simulink model "modelh"  (R2019b)
settings: Solver=VariableStepAuto  StartTime=0.0  StopTime=10.0  RelTol=1e-3
values from neighbouring files (symbols this model uses):
  alphaH = 1-exp(-1/d_Hj)    [parameters.m]
  alphaI = 1-exp(-d_Is)    [parameters.m]
  alphaJ = 1-exp(-1/d_J)    [parameters.m]
  beta_h = 0.66    [parameters.m]
  beta_l = 0.01    [parameters.m]
  c = 2    [parameters.m]
  gammaA = 1-exp(-1/d_Ia)    [parameters.m]
  gammaH = 1-exp(-1/d_Hr)    [parameters.m]
  gammaZ = 1-exp(-1/d_Iz)    [parameters.m]
  p_d_mu = 0.49    [parameters.m]
  p_d_sd = 0.1    [parameters.m]
  p_h = 0.055    [parameters.m]
  p_j_mu = 0.23    [parameters.m]
  p_j_sd = 0.1    [parameters.m]
  p_s_h = 0.99    [parameters.m]
  p_s_l = 0.5    [parameters.m]
  psi = 1-exp(-1/d_Ip)    [parameters.m]
  r_beta_h = 0.99    [parameters.m]
  r_beta_l = 0.4    [parameters.m]
  r_c_h = 0.5    [parameters.m]
  r_c_l = 0.01    [parameters.m]
  sigma = 1 - exp(-1/d_E)    [parameters.m]
settings Model: Creator=Viktor  LastModifiedBy=Viktor

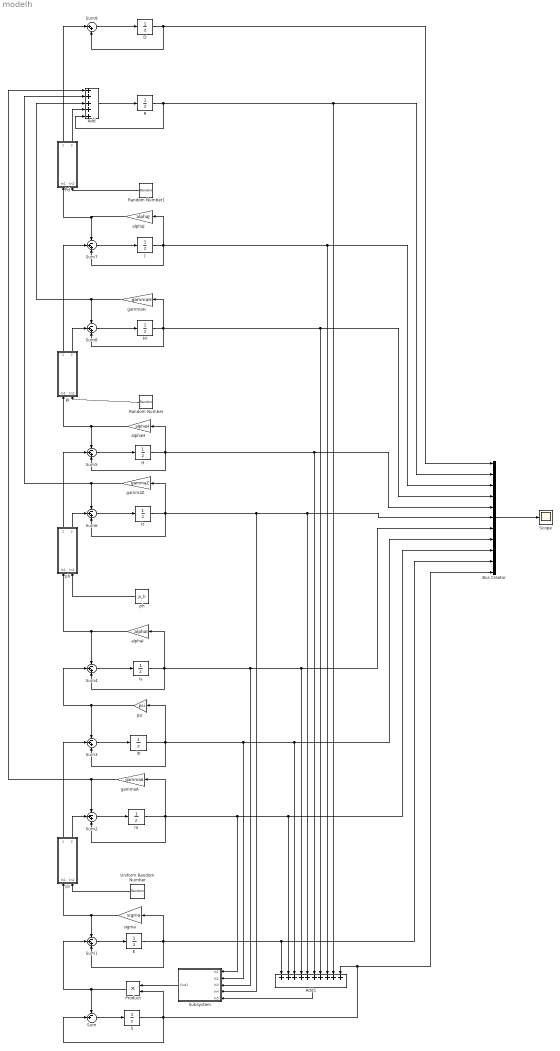
== system modelh ==
  Add : Sum  Inputs=+++++
  Add1 : Sum  Inputs=++++++++++
  Bus Creator : BusCreator  Inputs=11
  D : UnitDelay  SampleTime=-1  HasFrameUpgradeWarning=on
  E : UnitDelay  InitialCondition=10000  SampleTime=-1  HasFrameUpgradeWarning=on
  H : UnitDelay  InitialCondition=5000  SampleTime=-1  HasFrameUpgradeWarning=on
  Hr : UnitDelay  InitialCondition=5000  SampleTime=-1  HasFrameUpgradeWarning=on
  Ia : UnitDelay  InitialCondition=5000  SampleTime=-1  HasFrameUpgradeWarning=on
  Ip : UnitDelay  InitialCondition=5000  SampleTime=-1  HasFrameUpgradeWarning=on
  Is : UnitDelay  InitialCondition=5000  SampleTime=-1  HasFrameUpgradeWarning=on
  Iz : UnitDelay  InitialCondition=5000  SampleTime=-1  HasFrameUpgradeWarning=on
  J : UnitDelay  InitialCondition=5000  SampleTime=-1  HasFrameUpgradeWarning=on
  Pd : Subsystem
  Product : Product
  R : UnitDelay  InitialCondition=5000  SampleTime=-1  HasFrameUpgradeWarning=on
  Random Number : RandomNumber  Mean=p_j_mu  Variance=p_j_sd  SampleTime=0.1
  Random Number1 : RandomNumber  Mean=p_d_mu  Variance=p_d_sd  SampleTime=0.1
  S : UnitDelay  InitialCondition=5000000  SampleTime=-1  HasFrameUpgradeWarning=on
  Scope : Scope
  Subsystem : Subsystem
  Sum : Sum  Inputs=-+|
  Sum{1..8} (8 alike) : Sum  Inputs=-++
  Sum9 : Sum  Inputs=|++
  Uniform Random Number : UniformRandomNumber  Minimum=p_s_l  Maximum=p_s_h  SampleTime=0.1
  alphaH : Gain  Gain=alphaH
  alphaI : Gain  Gain=alphaI
  alphaJ : Gain  Gain=alphaJ
  gammaA : Gain  Gain=gammaA
  gammaH : Gain  Gain=gammaH
  gammaZ : Gain  Gain=gammaZ
  ph : Subsystem
  "ph " : Constant  Value=p_h
  pj : Subsystem
  "ps " : Subsystem
  psi : Gain  Gain=psi
  sigma : Gain  Gain=sigma
  wires:
  S/1 -> Product/2, Bus Creator/11, Add1/10, Sum/2
  Sum/1 -> S/1
  Product/1 -> Sum1/2, Sum/1
  Sum1/1 -> E/1
  sigma/1 -> Sum1/1, "ps "/1(In1)
  Uniform Random Number/1 -> "ps "/2(In2)
  "ps "/2(Out2) -> Sum2/2
  Sum2/1 -> Ia/1
  Ia/1 -> Subsystem/1(In1), Bus Creator/9, Add1/2, gammaA/1, Sum2/3
  Sum3/1 -> Ip/1
  Ip/1 -> Subsystem/2(In2), Bus Creator/8, Add1/3, psi/1, Sum3/3
  "ps "/1(Out1) -> Sum3/2
  psi/1 -> Sum4/2, Sum3/1
  Sum4/1 -> Is/1
  Is/1 -> Subsystem/3(In3), Bus Creator/7, Add1/4, alphaI/1, Sum4/3
  alphaI/1 -> ph/1(In1), Sum4/1
  "ph "/1 -> ph/2(In2)
  Sum5/1 -> H/1
  alphaH/1 -> pj/1(In1), Sum5/1
  Sum6/1 -> Iz/1
  Iz/1 -> Add1/5, Bus Creator/6, Subsystem/4(In4), gammaZ/1, Sum6/3
  ph/2(Out2) -> Sum6/2
  gammaZ/1 -> Add/2, Sum6/1
  Sum7/1 -> J/1
  Random Number/1 -> pj/2(In2)
  pj/1(Out1) -> Sum7/2
  Sum8/1 -> Hr/1
  pj/2(Out2) -> Sum8/2
  gammaH/1 -> Sum8/1, Add/3
  alphaJ/1 -> Pd/1(In1), Sum7/1
  Random Number1/1 -> Pd/2(In2)
  Pd/1(Out1) -> Sum9/1
  Sum9/1 -> D/1
  D/1 -> Sum9/2, Bus Creator/1
  Add/1 -> R/1
  Pd/2(Out2) -> Add/4
  ph/1(Out1) -> Sum5/2
  gammaA/1 -> Sum2/1, Add/1
  Add1/1 -> Subsystem/5(In5)
  Subsystem/1(Out1) -> Product/1
  R/1 -> Bus Creator/2, Add1/9, Add/5
  J/1 -> Add1/8, Bus Creator/3, alphaJ/1, Sum7/3
  Hr/1 -> Add1/7, Bus Creator/4, gammaH/1, Sum8/3
  H/1 -> Add1/6, Bus Creator/5, alphaH/1, Sum5/3
  E/1 -> Bus Creator/10, Add1/1, sigma/1, Sum1/3
  Bus Creator/1 -> Scope/1

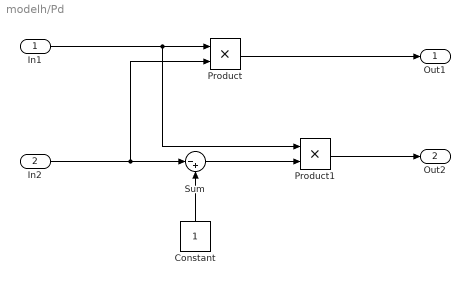
== system modelh/Pd ==
  In1 : Inport
  In2 : Inport  Port=2
  Constant : Constant
  Product : Product
  Product1 : Product
  Sum : Sum  Inputs=|-+
  Out1 : Outport
  Out2 : Outport  Port=2
  wires:
  In1/1 -> Product1/1, Product/1
  Product/1 -> Out1/1
  In2/1 -> Sum/1, Product/2
  Constant/1 -> Sum/2
  Sum/1 -> Product1/2
  Product1/1 -> Out2/1

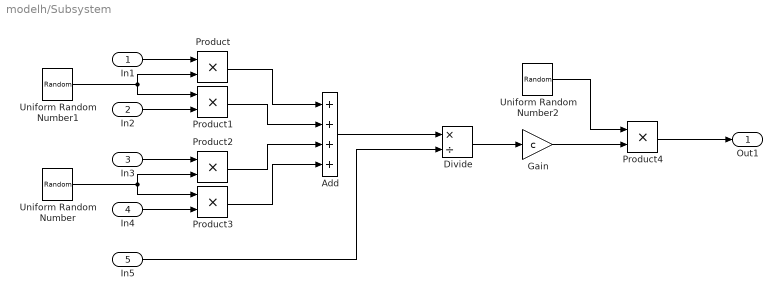
== system modelh/Subsystem ==
  In1 : Inport
  In2 : Inport  Port=2
  In3 : Inport  Port=3
  In4 : Inport  Port=4
  In5 : Inport  Port=5
  Add : Sum  Inputs=++++
  Divide : Product  Inputs=*/
  Gain : Gain  Gain=c
  Product{,1..4} (5 alike) : Product
  Uniform Random Number : UniformRandomNumber  Minimum=r_c_l  Maximum=r_c_h  SampleTime=0.1
  Uniform Random Number1 : UniformRandomNumber  Minimum=r_beta_l  Maximum=r_beta_h  SampleTime=0.1
  Uniform Random Number2 : UniformRandomNumber  Minimum=beta_l  Maximum=beta_h  SampleTime=0.1
  Out1 : Outport
  wires:
  In1/1 -> Product/1
  In2/1 -> Product1/2
  In3/1 -> Product2/1
  In4/1 -> Product3/2
  Uniform Random Number/1 -> Product3/1, Product2/2
  Uniform Random Number1/1 -> Product1/1, Product/2
  Product1/1 -> Add/2
  Product2/1 -> Add/3
  Product3/1 -> Add/4
  Product/1 -> Add/1
  Add/1 -> Divide/1
  In5/1 -> Divide/2
  Divide/1 -> Gain/1
  Gain/1 -> Product4/2
  Product4/1 -> Out1/1
  Uniform Random Number2/1 -> Product4/1

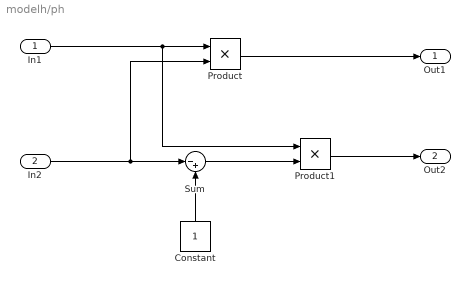
== system modelh/ph ==
  In1 : Inport
  In2 : Inport  Port=2
  Constant : Constant
  Product : Product
  Product1 : Product
  Sum : Sum  Inputs=|-+
  Out1 : Outport
  Out2 : Outport  Port=2
  wires:
  In1/1 -> Product1/1, Product/1
  Product/1 -> Out1/1
  In2/1 -> Sum/1, Product/2
  Constant/1 -> Sum/2
  Sum/1 -> Product1/2
  Product1/1 -> Out2/1

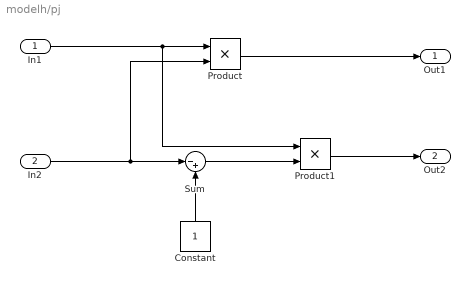
== system modelh/pj ==
  In1 : Inport
  In2 : Inport  Port=2
  Constant : Constant
  Product : Product
  Product1 : Product
  Sum : Sum  Inputs=|-+
  Out1 : Outport
  Out2 : Outport  Port=2
  wires:
  In1/1 -> Product1/1, Product/1
  Product/1 -> Out1/1
  In2/1 -> Sum/1, Product/2
  Constant/1 -> Sum/2
  Sum/1 -> Product1/2
  Product1/1 -> Out2/1

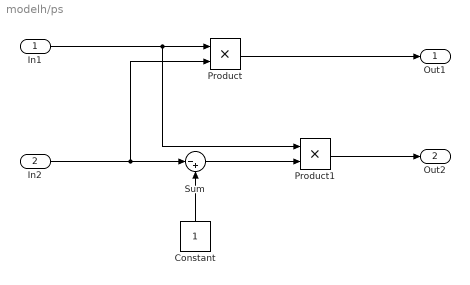
== system modelh/ps  ==
  In1 : Inport
  In2 : Inport  Port=2
  Constant : Constant
  Product : Product
  Product1 : Product
  Sum : Sum  Inputs=|-+
  Out1 : Outport
  Out2 : Outport  Port=2
  wires:
  In1/1 -> Product1/1, Product/1
  Product/1 -> Out1/1
  In2/1 -> Sum/1, Product/2
  Constant/1 -> Sum/2
  Sum/1 -> Product1/2
  Product1/1 -> Out2/1
